simulink model "modello_nave"  (R2023b)
settings: Solver=VariableStepAuto  StartTime=0.0  StopTime=10.0  RelTol=1e-3
values from neighbouring files (symbols this model uses):
  phi_0 = 0    [parametri.m]    (also in prova_matrici_jaco.m)
  r_0 = 0    [parametri.m]    (also in prova_matrici_jaco.m)
  tau_r_0 = 0    [parametri.m]    (also in prova_matrici_jaco.m)
  tau_u_0 = 0    [parametri.m]    (also in prova_matrici_jaco.m)
  u_0 = 0    [parametri.m]    (also in prova_matrici_jaco.m)
  v_0 = 0    [parametri.m]    (also in prova_matrici_jaco.m)
  x_0 = 0    [parametri.m]    (also in prova_matrici_jaco.m)
  y_0 = 0    [parametri.m]    (also in prova_matrici_jaco.m)
settings Model: Creator=edoca  LastModifiedBy=edoca

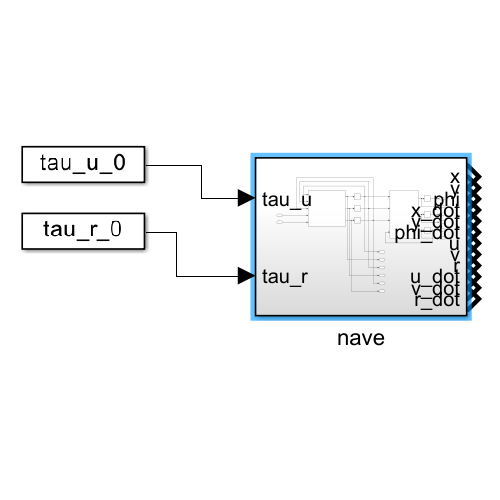
[thumbnail: Simulink's stored preview of the top-level diagram]
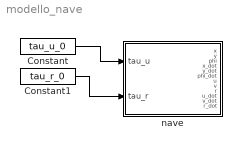
== system modello_nave ==
  Constant : Constant  Value=tau_u_0
  Constant1 : Constant  Value=tau_r_0
  nave : Subsystem
  wires:
  Constant/1 -> nave/1(tau_u)
  Constant1/1 -> nave/2(tau_r)

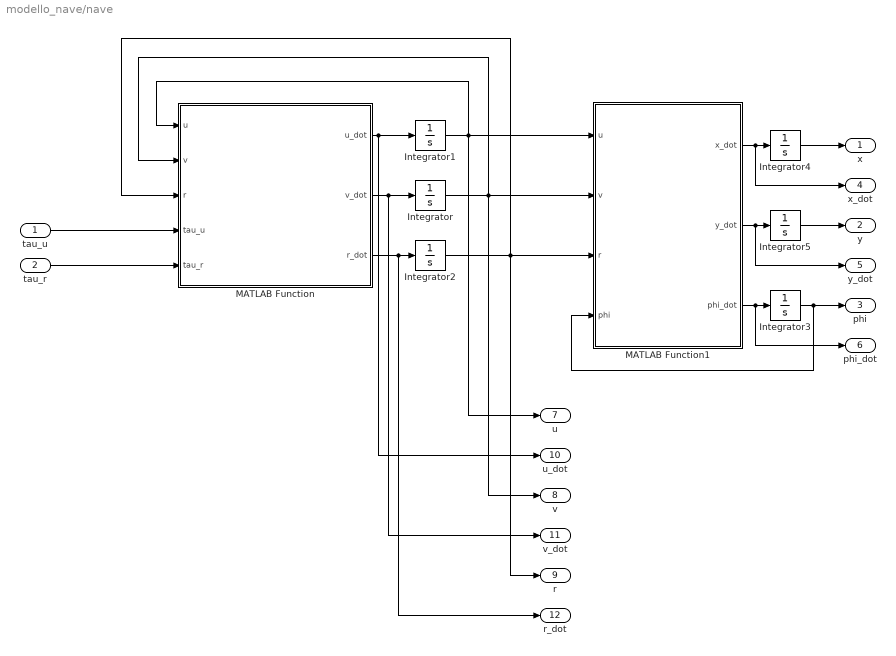
== system modello_nave/nave ==
  tau_u : Inport
  tau_r : Inport  Port=2
  Integrator : Integrator  InitialCondition=v_0
  Integrator1 : Integrator  InitialCondition=u_0
  Integrator2 : Integrator  InitialCondition=r_0
  Integrator3 : Integrator  InitialCondition=phi_0
  Integrator4 : Integrator  InitialCondition=x_0
  Integrator5 : Integrator  InitialCondition=y_0
  MATLAB Function : MATLAB Function  TreatAsAtomicUnit=on
  MATLAB Function1 : MATLAB Function  TreatAsAtomicUnit=on
  x : Outport
  y : Outport  Port=2
  phi : Outport  Port=3
  x_dot : Outport  Port=4
  y_dot : Outport  Port=5
  phi_dot : Outport  Port=6
  u : Outport  Port=7
  v : Outport  Port=8
  r : Outport  Port=9
  u_dot : Outport  Port=10
  v_dot : Outport  Port=11
  r_dot : Outport  Port=12
  wires:
  tau_r/1 -> MATLAB Function/5(tau_r)
  MATLAB Function1/1(x_dot) -> x_dot/1, Integrator4/1
  Integrator3/1 -> phi/1, MATLAB Function1/4(phi)
  Integrator4/1 -> x/1
  Integrator1/1 -> u/1, MATLAB Function1/1(u), MATLAB Function/1(u)
  MATLAB Function/3(r_dot) -> r_dot/1, Integrator2/1
  Integrator2/1 -> r/1, MATLAB Function/3(r), MATLAB Function1/3(r)
  MATLAB Function/2(v_dot) -> Integrator/1, v_dot/1
  Integrator5/1 -> y/1
  MATLAB Function1/3(phi_dot) -> phi_dot/1, Integrator3/1
  Integrator/1 -> v/1, MATLAB Function/2(v), MATLAB Function1/2(v)
  tau_u/1 -> MATLAB Function/4(tau_u)
  MATLAB Function/1(u_dot) -> Integrator1/1, u_dot/1
  MATLAB Function1/2(y_dot) -> y_dot/1, Integrator5/1

== matlab function modello_nave/nave/MATLAB Function1 ==
  data: u input; x_dot output; v input; r input; phi input; y_dot output; phi_dot output
function [x_dot, y_dot, phi_dot] = state_dynamic(u, v, r, phi)

    x_dot = u*cos(phi) - v*sin(phi);
    y_dot = u*sin(phi) + v*cos(phi);
    phi_dot = r;

end

== matlab function modello_nave/nave/MATLAB Function ==
  data: u input; u_dot output; v input; r input; tau_u input; tau_r input; v_dot output; r_dot output; params parameter
function [u_dot, v_dot, r_dot] = velocity_dynamic(u, v, r, tau_u, tau_r, params)
    
    m11 = params(1);
    m22 = params(2);
    m33 = params(3);

    d11 = params(4);
    d22 = params(5);
    d33 = params(6);

    u_dot = (m22/m11)*v*r - (d11/m11)*u + (1/m11)*tau_u;
    v_dot = -(m11/m22)*u*r - (d22/m22)*v;
    r_dot = ((m11 - m22)/m33)*u*v - (d33/m33)*r + (1/m33)*tau_r;

end
